simulink model "step_size"  (Simulink 6.4)
settings: Solver=ode1  StartTime=0.0  StopTime=10  FixedStep=.01  RelTol=1e-3
libraries: simulink x1
settings Model: LastModifiedBy=C09Shankar.Kulumani

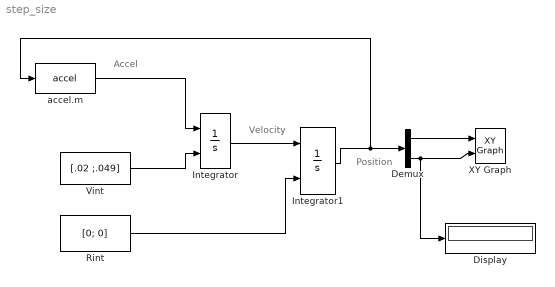
== system step_size ==
  note: Accel
  note: Velocity
  note: Position
  Demux : Demux  Outputs=2
  Display : Display
      settings: Format=short_e
  Integrator : Integrator  InitialConditionSource=external
  Integrator1 : Integrator  InitialConditionSource=external
  Rint : Constant  Value=[0; 0]  VectorParams1D=off  OutDataType=sfix(16)  ConRadixGroup=Use specified scaling  OutScaling=2^0  SampleTime=inf  FramePeriod=inf
  Vint : Constant  Value=[.02 ;.049]  VectorParams1D=off  OutDataType=sfix(16)  ConRadixGroup=Use specified scaling  OutScaling=2^0  SampleTime=inf  FramePeriod=inf
  XY Graph : simulink/Sinks/XY Graph  SystemSampleTime=-1  xmin=0  xmax=.2  ymin=0  ymax=.2  st=-1
  accel.m : MATLABFcn  MATLABFcn=accel  Output1D=off
  wires:
  accel.m/1 -> Integrator/1
  Vint/1 -> Integrator/2
  Rint/1 -> Integrator1/2
  Integrator/1 -> Integrator1/1
  Integrator1/1 -> Demux/1, accel.m/1
  Demux/2 -> Display/1, XY Graph/2
  Demux/1 -> XY Graph/1
